simulink model "One_Solar_Cell_Modelling"  (R2014b)
settings: Solver=ode23tb  StartTime=0.0  StopTime=2  RelTol=1e-3
libraries: simulink x3
settings Model: Creator=Amr Saleh  LastModifiedBy=Amr Saleh

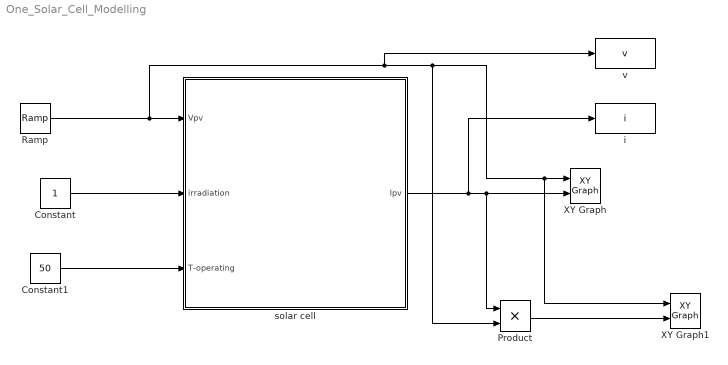
== system One_Solar_Cell_Modelling ==
  Constant : Constant
  Constant1 : Constant  Value=50
  Product : Product
  Ramp : simulink/Sources/Ramp  slope=22  start=0  X0=0
  XY Graph : simulink/Sinks/XY Graph  xmin=0  xmax=25  ymin=0  ymax=8  st=-1
  XY Graph1 : simulink/Sinks/XY Graph  xmin=0  xmax=25  ymin=0  ymax=70  st=-1
  i : ToWorkspace  VariableName=i  SampleTime=-1
  solar cell : Subsystem
  v : ToWorkspace  VariableName=v  SampleTime=-1
  wires:
  Constant/1 -> solar cell/2(irradiation)
  Constant1/1 -> solar cell/3(T-operating)
  Ramp/1 -> v/1, Product/2, XY Graph1/1, XY Graph/1, solar cell/1(Vpv)
  solar cell/1(Ipv) -> i/1, Product/1, XY Graph/2
  Product/1 -> XY Graph1/2

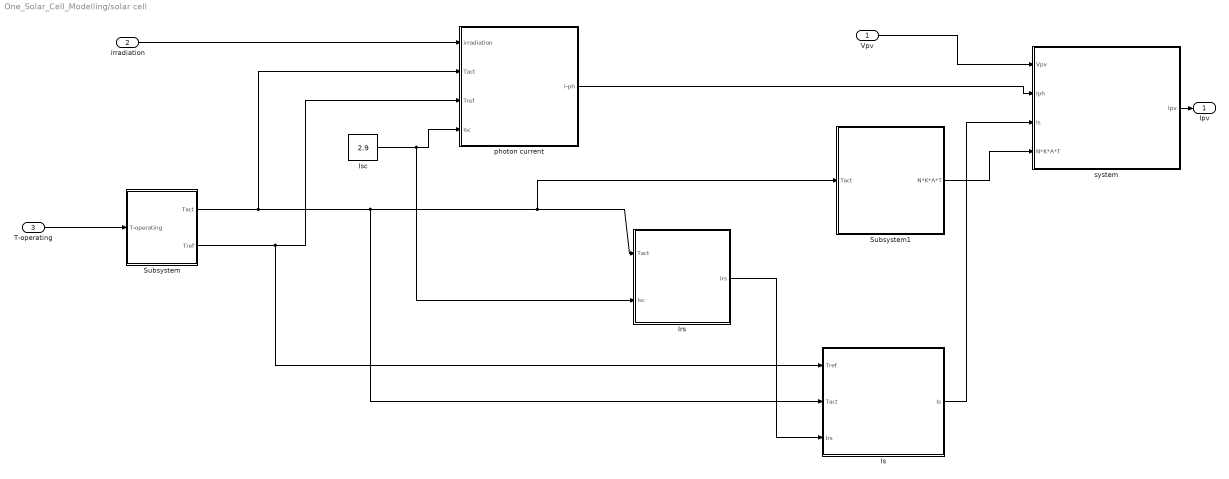
== system One_Solar_Cell_Modelling/solar cell ==
  Vpv : Inport
  irradiation : Inport  Port=2
  T-operating : Inport  Port=3
  Irs : Subsystem
  Is : Subsystem
  Isc : Constant  Value=2.9
  Subsystem : Subsystem
  Subsystem1 : Subsystem
  photon current : Subsystem
  system : Subsystem
  Ipv : Outport
  wires:
  Subsystem/1(Tact) -> photon current/2(Tact), Is/2(Tact), Subsystem1/1(Tact), Irs/1(Tact)
  Subsystem/2(Tref) -> Is/1(Tref), photon current/3(Tref)
  T-operating/1 -> Subsystem/1(T-operating)
  system/1(Ipv) -> Ipv/1
  Irs/1(Irs) -> Is/3(Irs)
  Subsystem1/1(N*K*A*T) -> system/4(N*K*A*T)
  irradiation/1 -> photon current/1(irradiation)
  Isc/1 -> Irs/2(Isc), photon current/4(Isc)
  Is/1(Is) -> system/3(Is)
  Vpv/1 -> system/1(Vpv)
  photon current/1(I-ph) -> system/2(Iph)

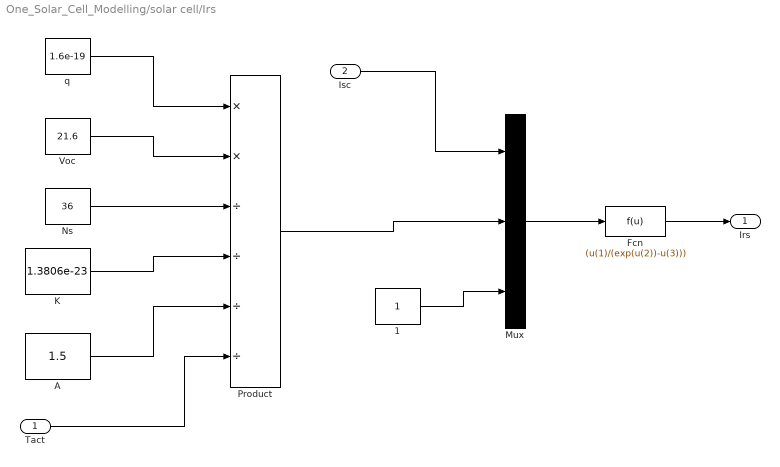
== system One_Solar_Cell_Modelling/solar cell/Irs ==
  Tact : Inport
  Isc : Inport  Port=2
  1 : Constant
  A : Constant  Value=1.5
  Fcn : Fcn  Expr=(u(1)/(exp(u(2))-u(3)))
  K : Constant  Value=1.3806e-23
  Mux : Mux  Inputs=3
  Ns : Constant  Value=36
  Product : Product  Inputs=**////
  Voc : Constant  Value=21.6
  q : Constant  Value=1.6e-19
  Irs : Outport
  wires:
  Mux/1 -> Fcn/1
  Ns/1 -> Product/3
  Voc/1 -> Product/2
  Tact/1 -> Product/6
  K/1 -> Product/4
  A/1 -> Product/5
  q/1 -> Product/1
  Fcn/1 -> Irs/1
  1/1 -> Mux/3
  Product/1 -> Mux/2
  Isc/1 -> Mux/1

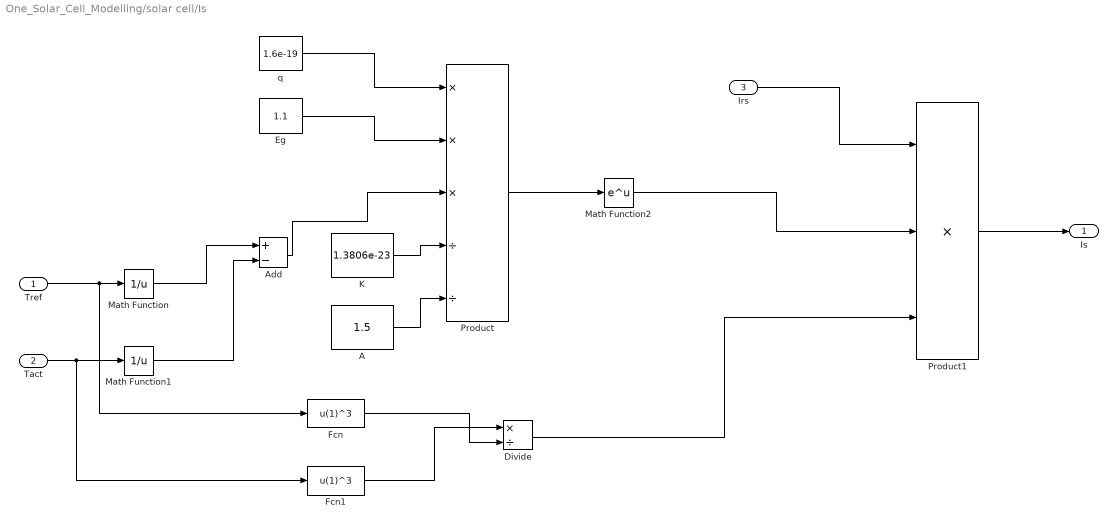
== system One_Solar_Cell_Modelling/solar cell/Is ==
  Tref : Inport
  Tact : Inport  Port=2
  Irs : Inport  Port=3
  A : Constant  Value=1.5
  Add : Sum  Inputs=+-
  Divide : Product  Inputs=*/
  Eg : Constant  Value=1.1
  Fcn : Fcn  Expr=u(1)^3
  Fcn1 : Fcn  Expr=u(1)^3
  K : Constant  Value=1.3806e-23
  Math Function : Math  Operator=reciprocal  SaturateOnIntegerOverflow=on
  Math Function1 : Math  Operator=reciprocal  SaturateOnIntegerOverflow=on
  Math Function2 : Math  SaturateOnIntegerOverflow=on
  Product : Product  Inputs=***//
  Product1 : Product  Inputs=***
  q : Constant  Value=1.6e-19
  Is : Outport
  wires:
  Eg/1 -> Product/2
  Fcn/1 -> Divide/2
  Tref/1 -> Fcn/1, Math Function/1
  q/1 -> Product/1
  Fcn1/1 -> Divide/1
  A/1 -> Product/5
  Divide/1 -> Product1/3
  Math Function1/1 -> Add/2
  Add/1 -> Product/3
  Math Function2/1 -> Product1/2
  Irs/1 -> Product1/1
  Math Function/1 -> Add/1
  K/1 -> Product/4
  Product/1 -> Math Function2/1
  Product1/1 -> Is/1
  Tact/1 -> Fcn1/1, Math Function1/1

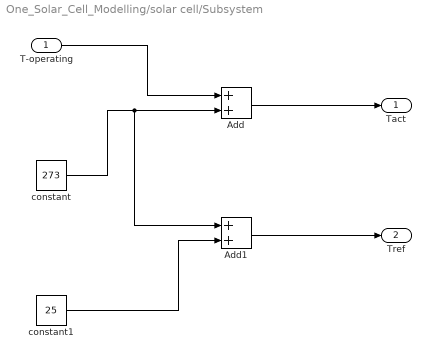
== system One_Solar_Cell_Modelling/solar cell/Subsystem ==
  T-operating : Inport
  Add : Sum
  Add1 : Sum
  constant : Constant  Value=273
  constant1 : Constant  Value=25
  Tact : Outport
  Tref : Outport  Port=2
  wires:
  Add1/1 -> Tref/1
  constant/1 -> Add1/1, Add/2
  Add/1 -> Tact/1
  T-operating/1 -> Add/1
  constant1/1 -> Add1/2

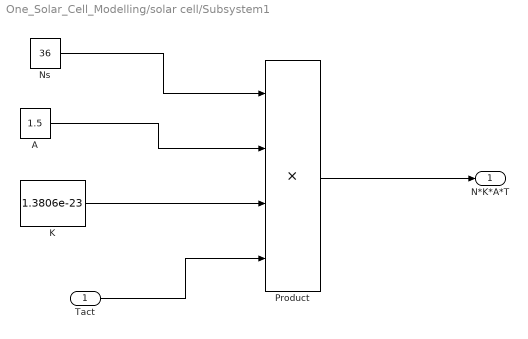
== system One_Solar_Cell_Modelling/solar cell/Subsystem1 ==
  Tact : Inport
  A : Constant  Value=1.5
  K : Constant  Value=1.3806e-23
  Ns : Constant  Value=36
  Product : Product  Inputs=****
  N*K*A*T : Outport
  wires:
  Tact/1 -> Product/4
  K/1 -> Product/3
  A/1 -> Product/2
  Product/1 -> N*K*A*T/1
  Ns/1 -> Product/1

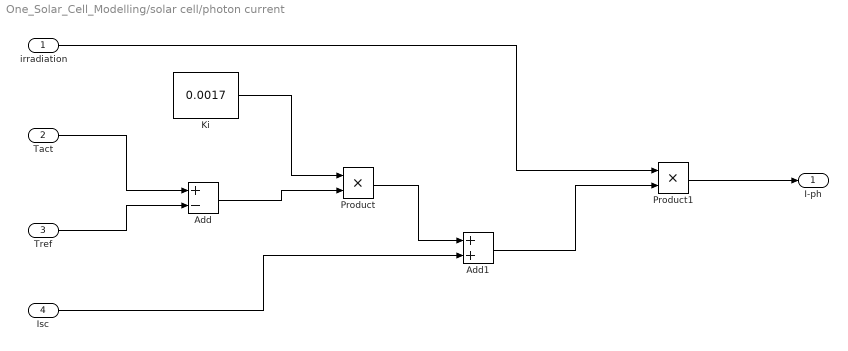
== system One_Solar_Cell_Modelling/solar cell/photon current ==
  irradiation : Inport
  Tact : Inport  Port=2
  Tref : Inport  Port=3
  Isc : Inport  Port=4
  Add : Sum  Inputs=+-
  Add1 : Sum
  Ki : Constant  Value=0.0017
  Product : Product
  Product1 : Product
  I-ph : Outport
  wires:
  Isc/1 -> Add1/2
  Product/1 -> Add1/1
  Add/1 -> Product/2
  Product1/1 -> I-ph/1
  Ki/1 -> Product/1
  Tact/1 -> Add/1
  Tref/1 -> Add/2
  irradiation/1 -> Product1/1
  Add1/1 -> Product1/2

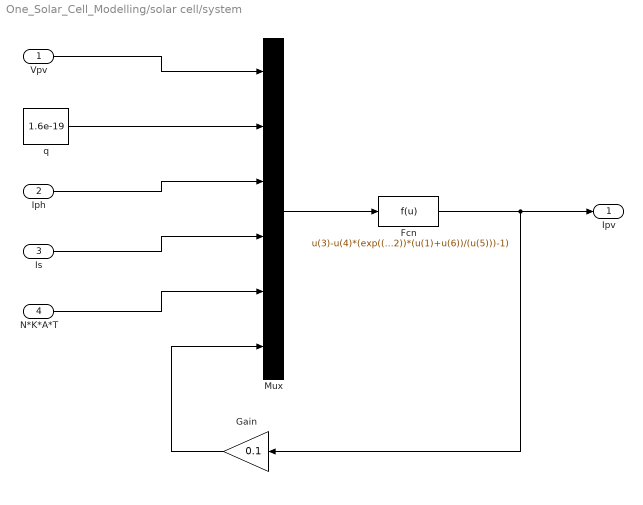
== system One_Solar_Cell_Modelling/solar cell/system ==
  Vpv : Inport
  Iph : Inport  Port=2
  Is : Inport  Port=3
  N*K*A*T : Inport  Port=4
  Fcn : Fcn  Expr=u(3)-u(4)*(exp((u(2))*(u(1)+u(6))/(u(5)))-1)
  Gain : Gain  Gain=0.1
  Mux : Mux  Inputs=6
  q : Constant  Value=1.6e-19
  Ipv : Outport
  wires:
  Mux/1 -> Fcn/1
  Iph/1 -> Mux/3
  q/1 -> Mux/2
  Fcn/1 -> Ipv/1, Gain/1
  Is/1 -> Mux/4
  N*K*A*T/1 -> Mux/5
  Vpv/1 -> Mux/1
  Gain/1 -> Mux/6
